simulink model "testingmodel"  (Simulink 8.7)
settings: Solver=VariableStepAuto  StartTime=0.0  StopTime=10.0  RelTol=1e-3
libraries: simulink x1
settings Model: Creator=pfj01  LastModifiedBy=pfj01
settings DataIOCC: LimitDataPoints=off  SaveFormat=Dataset
settings DebuggingCC: UnderspecifiedInitializationDetection=Simplified  MergeDetectMultiDrivingBlocksExec=error
settings HardwareCC: ProdBitPerPointer=64  ProdLargestAtomicFloat=Float  ProdIntDivRoundTo=Zero  ProdEndianess=LittleEndian  ProdWordSize=64  ProdHWDeviceType=Intel->x86-64 (Windows64)
settings ModelReferenceCC: PropagateSignalLabelsOutOfModel=on
settings ConfigComp: CovModelRefEnable=off

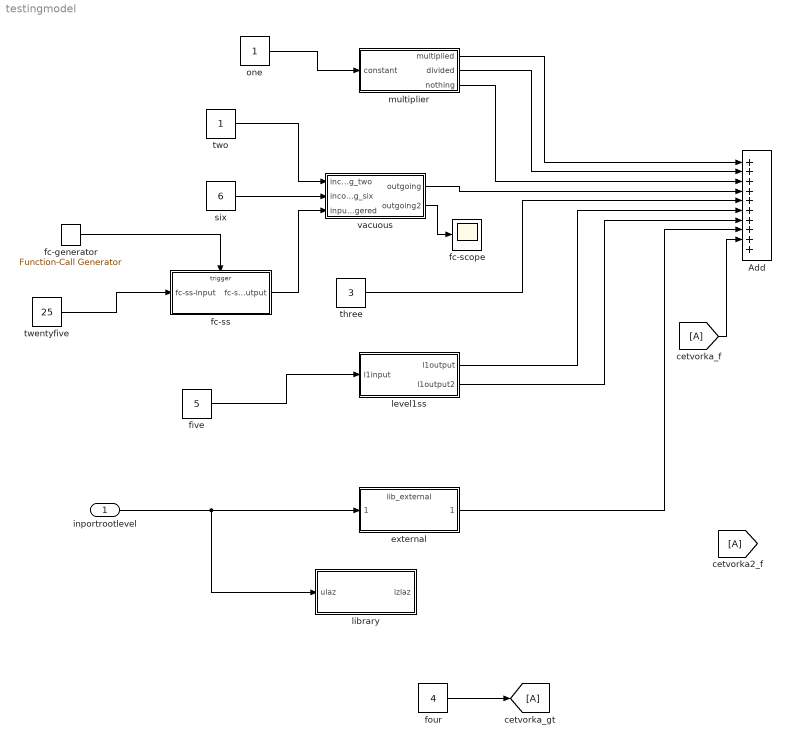
== system testingmodel ==
  inportrootlevel : Inport
  Add : Sum  Inputs=++++++++++
  external : ModelReference  ModelNameDialog=lib_external.mdl  SimulationMode=Normal  ModelReferenceVersion=1.11
  fc-generator : simulink/Ports & Subsystems/Function-Call Generator  sample_time=10  numberOfIterations=1
  fc-scope : Scope
  fc-ss : Subsystem  TreatAsAtomicUnit=on
  five : Constant  Value=5
  four : Constant  Value=4
  level1ss : Subsystem
  library : Subsystem  TreatAsAtomicUnit=on
  multiplier : Subsystem
  one : Constant
  six : Constant  Value=6
  three : Constant  Value=3
  twentyfive : Constant  Value=25
  two : Constant
  vacuous : Subsystem
  wires:
  one/1 -> multiplier/1(constant)
  multiplier/1(multiplied) -> Add/1
  two/1 -> vacuous/1(incoming_two)
  three/1 -> Add/5
  multiplier/2(divided) -> Add/2
  vacuous/1(outgoing) -> Add/4
  multiplier/3(nothing) -> Add/3
  level1ss/1(l1output) -> Add/6
  five/1 -> level1ss/1(l1input)
  level1ss/2(l1output2) -> Add/7
  inportrootlevel/1 -> library/1(ulaz), external/1
  external/1 -> Add/8
  six/1 -> vacuous/2(incoming_six)
  four/1 -> [A]
  [A] -> Add/9
  fc-ss/1(fc-ss-output) -> vacuous/3(input_triggered)
  fc-generator/1 -> fc-ss/Trigger
  twentyfive/1 -> fc-ss/1(fc-ss-input)
  vacuous/2(outgoing2) -> fc-scope/1

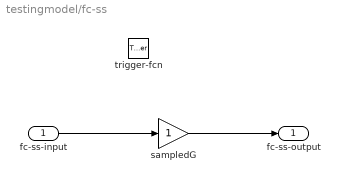
== system testingmodel/fc-ss ==
  fc-ss-input : Inport
  trigger-fcn : TriggerPort  TriggerType=function-call  VariantControl=Variant
  sampledG : Gain
  fc-ss-output : Outport
  wires:
  fc-ss-input/1 -> sampledG/1
  sampledG/1 -> fc-ss-output/1

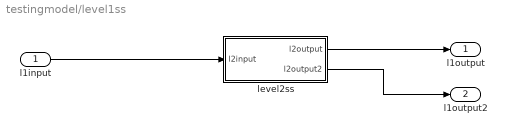
== system testingmodel/level1ss ==
  l1input : Inport
  level2ss : Subsystem
  l1output : Outport
  l1output2 : Outport  Port=2
  wires:
  l1input/1 -> level2ss/1(l2input)
  level2ss/1(l2output) -> l1output/1
  level2ss/2(l2output2) -> l1output2/1

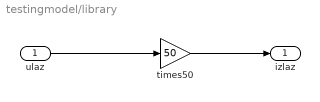
== system testingmodel/library ==
  ulaz : Inport
  times50 : Gain  Gain=50
  izlaz : Outport
  wires:
  ulaz/1 -> times50/1
  times50/1 -> izlaz/1

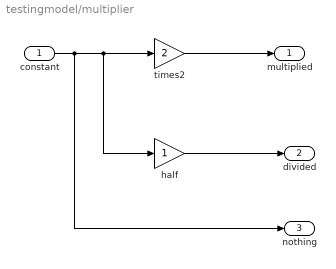
== system testingmodel/multiplier ==
  constant : Inport
  "half " : Gain
  times2 : Gain  Gain=2
  multiplied : Outport
  divided : Outport  Port=2
  nothing : Outport  Port=3
  wires:
  constant/1 -> nothing/1, "half "/1, times2/1
  times2/1 -> multiplied/1
  "half "/1 -> divided/1

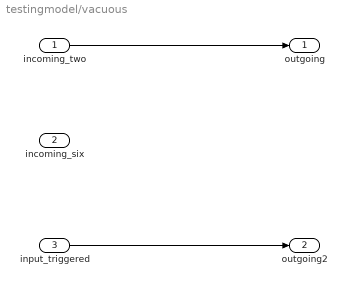
== system testingmodel/vacuous ==
  incoming_two : Inport
  incoming_six : Inport  Port=2
  input_triggered : Inport  Port=3
  outgoing : Outport
  outgoing2 : Outport  Port=2
  wires:
  incoming_two/1 -> outgoing/1
  input_triggered/1 -> outgoing2/1

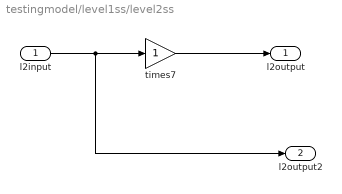
== system testingmodel/level1ss/level2ss ==
  l2input : Inport
  times7 : Gain
  l2output : Outport
  l2output2 : Outport  Port=2
  wires:
  l2input/1 -> l2output2/1, times7/1
  times7/1 -> l2output/1
